simulink model "untitled"  (R2018a)
settings: Solver=VariableStepAuto  StartTime=0.0  StopTime=10.0  RelTol=1e-3
settings Model: Creator=kyniu  LastModifiedBy=kyniu

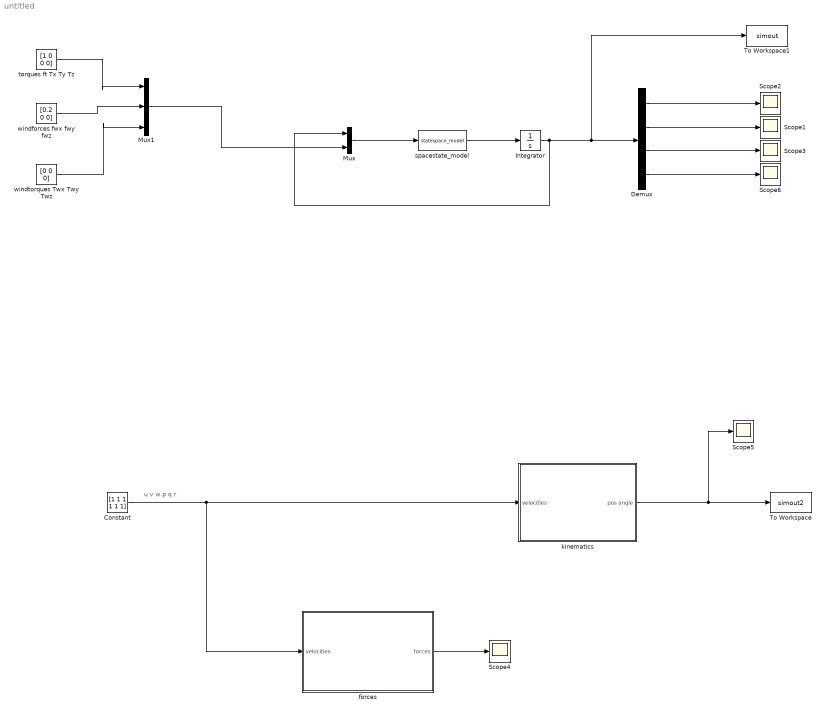
== system untitled ==
  note: u v w p q r
  Constant : Constant  Value=[1 1 1 1 1 1]
  Demux : Demux  Outputs=[3 3 3 3]
  Integrator : Integrator  InitialCondition=[0 0 0 0 0 0 0 0 0 0 0 0]
  Mux : Mux  Inputs=2
  Mux1 : Mux  Inputs=3
  Scope{1..6} (6 alike) : Scope
  To Workspace : ToWorkspace  VariableName=simout2  SaveFormat=Timeseries  SampleTime=-1
  To Workspace1 : ToWorkspace  VariableName=simout  SaveFormat=Timeseries  SampleTime=-1
  forces : Subsystem
  kinematics : Subsystem
  spacestate_model : MATLABFcn  MATLABFcn=statespace_model
  torques ft Tx Ty Tz : Constant  Value=[1 0 0 0]
  "windforces fwx fwy fwz " : Constant  Value=[0.2 0 0]
  windtorques Twx Twy Twz : Constant  Value=[0 0 0]
  wires:
  Constant/1 -> forces/1(velocities), kinematics/1(velocities)
  kinematics/1(pos angle) -> Scope5/1, To Workspace/1
  forces/1("forces ") -> Scope4/1
  spacestate_model/1 -> Integrator/1
  Integrator/1 -> To Workspace1/1, Demux/1, Mux/1
  Mux/1 -> spacestate_model/1
  torques ft Tx Ty Tz/1 -> Mux1/1
  "windforces fwx fwy fwz "/1 -> Mux1/2
  windtorques Twx Twy Twz/1 -> Mux1/3
  Mux1/1 -> Mux/2
  Demux/1 -> Scope2/1
  Demux/2 -> Scope1/1
  Demux/3 -> Scope3/1
  Demux/4 -> Scope6/1

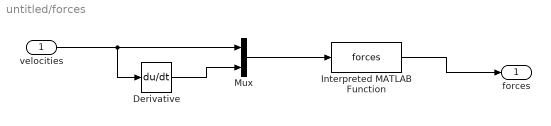
== system untitled/forces ==
  velocities : Inport
  Derivative : Derivative  CoefficientInTFapproximation=1
  Interpreted MATLAB Function : MATLABFcn  MATLABFcn=forces
  Mux : Mux  Inputs=2
  "forces " : Outport
  wires:
  velocities/1 -> Derivative/1, Mux/1
  Derivative/1 -> Mux/2
  Interpreted MATLAB Function/1 -> "forces "/1
  Mux/1 -> Interpreted MATLAB Function/1

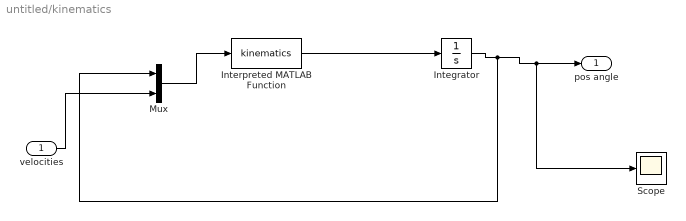
== system untitled/kinematics ==
  velocities : Inport
  Integrator : Integrator  InitialCondition=[0 0 0 0 0 0]
  Interpreted MATLAB Function : MATLABFcn  MATLABFcn=kinematics
  Mux : Mux  Inputs=[6 6]
  Scope : Scope
  pos angle : Outport
  wires:
  Mux/1 -> Interpreted MATLAB Function/1
  Integrator/1 -> Mux/1, pos angle/1, Scope/1
  velocities/1 -> Mux/2
  Interpreted MATLAB Function/1 -> Integrator/1
